simulink model "project_2_simulink"  (R2023b)
settings: Solver=VariableStepAuto  StartTime=0.0  StopTime=10.0  RelTol=1e-3
undefined symbols (not defined in the file or in its folder): k
settings Model: Creator=robertgraham  LastModifiedBy=robertgraham

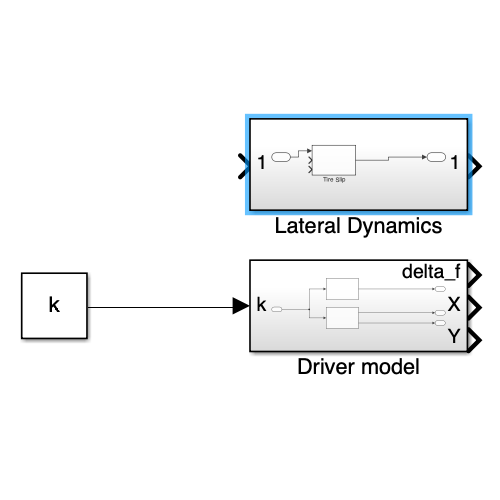
[thumbnail: Simulink's stored preview of the top-level diagram]
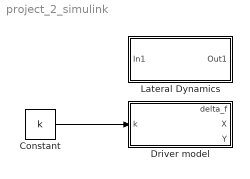
== system project_2_simulink ==
  Constant : Constant  Value=k
  Driver model : Subsystem
  Lateral Dynamics : Subsystem
  wires:
  Constant/1 -> Driver model/1(k)

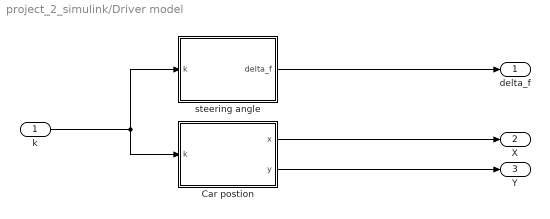
== system project_2_simulink/Driver model ==
  k : Inport
  "Car postion " : MATLAB Function  TreatAsAtomicUnit=on
  steering angle : MATLAB Function  TreatAsAtomicUnit=on
  delta_f : Outport
  X : Outport  Port=2
  Y : Outport  Port=3
  wires:
  k/1 -> "Car postion "/1(k), steering angle/1(k)
  steering angle/1(delta_f) -> delta_f/1
  "Car postion "/1(x) -> X/1
  "Car postion "/2(y) -> Y/1

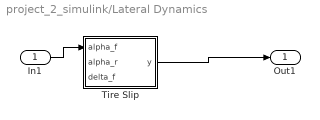
== system project_2_simulink/Lateral Dynamics ==
  In1 : Inport
  " Tire Slip" : MATLAB Function  TreatAsAtomicUnit=on
  Out1 : Outport
  wires:
  In1/1 -> " Tire Slip"/1(alpha_f)
  " Tire Slip"/1(y) -> Out1/1

== matlab function project_2_simulink/Driver model/steering angle ==
  data: k input; delta_f output
function delta_f = fcn(k)

% find delta_f steering angle
% input should be X and Y value

delta_f = atan2(yc(k)-yp(k),xc(k)- xp(k));

== matlab function project_2_simulink/Lateral Dynamics/ Tire Slip ==
  data: alpha_f input; y output; alpha_r input; delta_f input
function y = fcn(alpha_f,alpha_r,delta_f)

alpha_f = delta_f - atan2(vy+lf*omega,vx)

y = u;

== matlab function project_2_simulink/Driver model/Car postion  ==
  data: k input; x output; y output
function [x,y] = fcn(k)

% find delta_f steering angle
% input should be X and Y value

x = xc(k);
y = yc(k);
